simulink library "AtomicLibrary"
PostLoadFcn:
  | PacketBusGenerator
libraries: LinkLayer5 x2

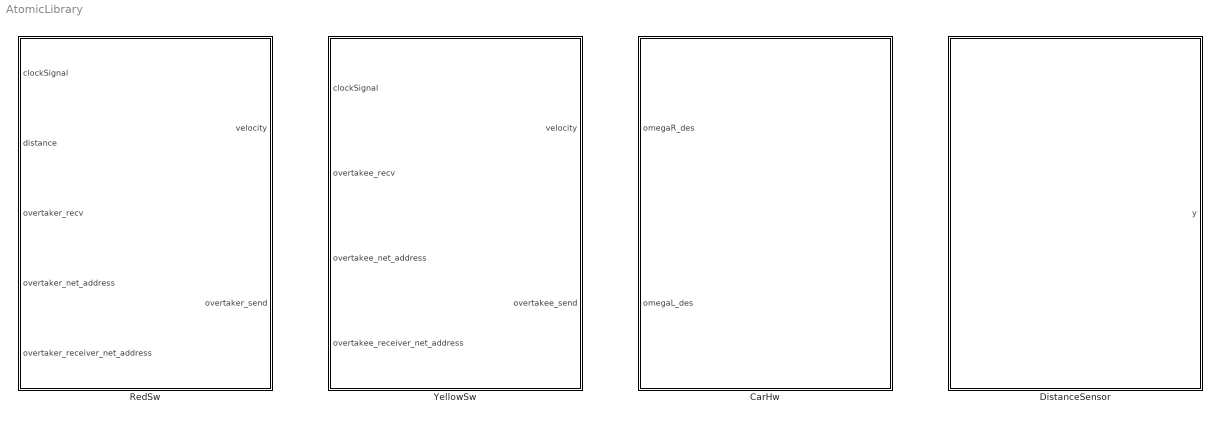
== system AtomicLibrary ==
  RedSw : Subsystem  Tag=id=_73wJYPUnEeOqvInL61-gjw
  YellowSw : Subsystem  Tag=id=_74DEU_UnEeOqvInL61-gjw
  CarHw : Subsystem  Tag=id=_74WmUPUnEeOqvInL61-gjw
  DistanceSensor : Subsystem  Tag=id=_74WmUfUnEeOqvInL61-gjw

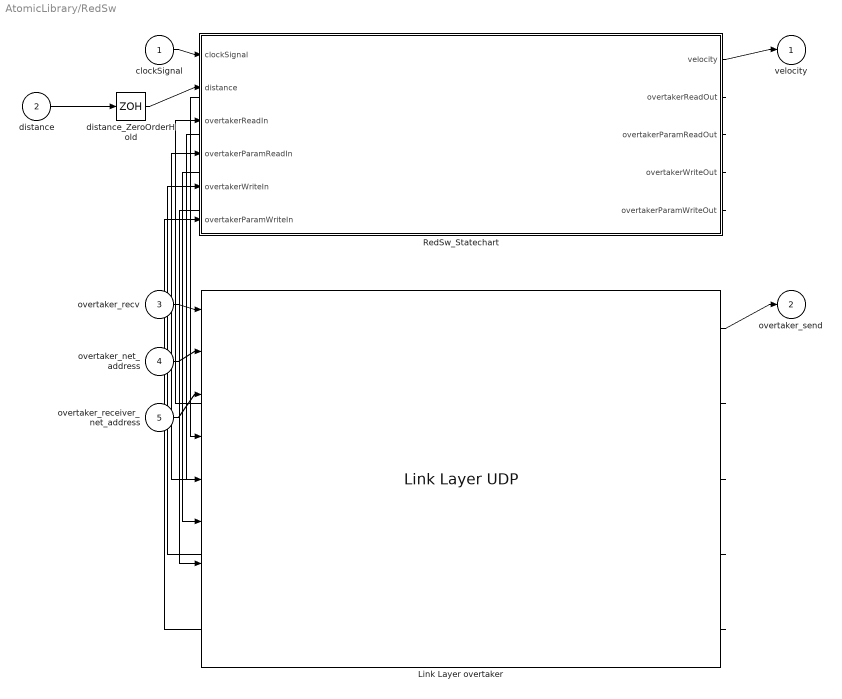
== system AtomicLibrary/RedSw ==
  clockSignal : Inport  Tag=id=_7356YvUnEeOqvInL61-gjw  Port=1  DataType=auto  OutDataType=fixdt(1, 16)  OutScaling=2^0  OutDataTypeStr=Inherit: auto
  distance : Inport  Tag=id=_77xGsPUnEeOqvInL61-gjw  Port=2  DataType=double  OutDataType=fixdt(1, 16)  OutScaling=2^0  OutDataTypeStr=double
  overtaker_recv : Inport  Tag=id=_780PkfUnEeOqvInL61-gjw  Port=3  DataType=auto  OutDataType=fixdt(1, 16)  OutScaling=2^0  UseBusObject=on  OutDataTypeStr=Inherit: auto
      settings: BusObject=PacketBus
  overtaker_net_address : Inport  Tag=id=_780Pk_UnEeOqvInL61-gjw  Port=4  DataType=uint8  OutDataType=fixdt(1, 16)  OutScaling=2^0  OutDataTypeStr=uint8
  overtaker_receiver_net_address : Inport  Tag=id=_780PlPUnEeOqvInL61-gjw  Port=5  DataType=uint8  OutDataType=fixdt(1, 16)  OutScaling=2^0  OutDataTypeStr=uint8
  velocity : Outport  Tag=id=_77VB0vUnEeOqvInL61-gjw  Port=1  DataType=double  OutDataType=fixdt(1, 16)  OutScaling=2^0  OutDataTypeStr=double
  overtaker_send : Outport  Tag=id=_780PkPUnEeOqvInL61-gjw  Port=2  DataType=auto  OutDataType=fixdt(1, 16)  OutScaling=2^0  UseBusObject=on  OutDataTypeStr=Inherit: auto
      settings: BusObject=PacketBus
  RedSw_Statechart : Stateflow chart  Tag=id=_73m_cPUnEeOqvInL61-gjw
  distance_ZeroOrderHold : ZeroOrderHold  Tag=id=_7763sPUnEeOqvInL61-gjw  SampleTime=30*0.001*1
  Link Layer overtaker : LinkLayer5/Link Layer UDP  DelayMin=1*1000  DelayMax=1*1000  MessageLossProbability=0  BufferOverflowPossible=on  SourceBufferSize=5  MessageMapping=[1 1; 2 1; 3 1; 4 1; 5 1]
  wires:
  clockSignal/1 -> RedSw_Statechart/1(clockSignal)
  RedSw_Statechart/1(velocity) -> velocity/1
  distance/1 -> distance_ZeroOrderHold/1
  distance_ZeroOrderHold/1 -> RedSw_Statechart/2(distance)
  Link Layer overtaker/1 -> overtaker_send/1
  overtaker_recv/1 -> Link Layer overtaker/1
  overtaker_net_address/1 -> Link Layer overtaker/2
  overtaker_receiver_net_address/1 -> Link Layer overtaker/3
  RedSw_Statechart/2(overtakerReadOut) -> Link Layer overtaker/4
  RedSw_Statechart/3(overtakerParamReadOut) -> Link Layer overtaker/5
  RedSw_Statechart/4(overtakerWriteOut) -> Link Layer overtaker/6
  RedSw_Statechart/5(overtakerParamWriteOut) -> Link Layer overtaker/7
  Link Layer overtaker/2 -> RedSw_Statechart/3(overtakerReadIn)
  Link Layer overtaker/3 -> RedSw_Statechart/4(overtakerParamReadIn)
  Link Layer overtaker/4 -> RedSw_Statechart/5(overtakerWriteIn)
  Link Layer overtaker/5 -> RedSw_Statechart/6(overtakerParamWriteIn)

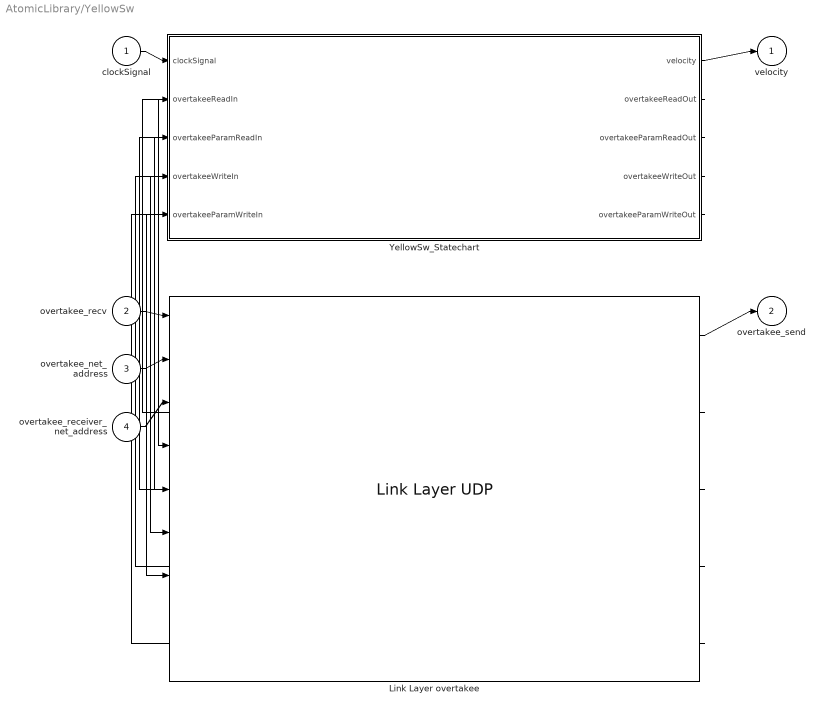
== system AtomicLibrary/YellowSw ==
  clockSignal : Inport  Tag=id=_74DEVvUnEeOqvInL61-gjw  Port=1  DataType=auto  OutDataType=fixdt(1, 16)  OutScaling=2^0  OutDataTypeStr=Inherit: auto
  overtakee_recv : Inport  Tag=id=_78gtlvUnEeOqvInL61-gjw  Port=2  DataType=auto  OutDataType=fixdt(1, 16)  OutScaling=2^0  UseBusObject=on  OutDataTypeStr=Inherit: auto
      settings: BusObject=PacketBus
  overtakee_net_address : Inport  Tag=id=_78gtmPUnEeOqvInL61-gjw  Port=3  DataType=uint8  OutDataType=fixdt(1, 16)  OutScaling=2^0  OutDataTypeStr=uint8
  overtakee_receiver_net_address : Inport  Tag=id=_78gtmfUnEeOqvInL61-gjw  Port=4  DataType=uint8  OutDataType=fixdt(1, 16)  OutScaling=2^0  OutDataTypeStr=uint8
  velocity : Outport  Tag=id=_77Bf0vUnEeOqvInL61-gjw  Port=1  DataType=double  OutDataType=fixdt(1, 16)  OutScaling=2^0  OutDataTypeStr=double
  overtakee_send : Outport  Tag=id=_78gtlfUnEeOqvInL61-gjw  Port=2  DataType=auto  OutDataType=fixdt(1, 16)  OutScaling=2^0  UseBusObject=on  OutDataTypeStr=Inherit: auto
      settings: BusObject=PacketBus
  YellowSw_Statechart : Stateflow chart  Tag=id=_74DEUfUnEeOqvInL61-gjw
  Link Layer overtakee : LinkLayer5/Link Layer UDP  DelayMin=1*1000  DelayMax=1*1000  MessageLossProbability=0  BufferOverflowPossible=on  SourceBufferSize=5  MessageMapping=[1 1; 2 1; 3 1; 4 1; 5 1]
  wires:
  clockSignal/1 -> YellowSw_Statechart/1(clockSignal)
  YellowSw_Statechart/1(velocity) -> velocity/1
  Link Layer overtakee/1 -> overtakee_send/1
  overtakee_recv/1 -> Link Layer overtakee/1
  overtakee_net_address/1 -> Link Layer overtakee/2
  overtakee_receiver_net_address/1 -> Link Layer overtakee/3
  YellowSw_Statechart/2(overtakeeReadOut) -> Link Layer overtakee/4
  YellowSw_Statechart/3(overtakeeParamReadOut) -> Link Layer overtakee/5
  YellowSw_Statechart/4(overtakeeWriteOut) -> Link Layer overtakee/6
  YellowSw_Statechart/5(overtakeeParamWriteOut) -> Link Layer overtakee/7
  Link Layer overtakee/2 -> YellowSw_Statechart/2(overtakeeReadIn)
  Link Layer overtakee/3 -> YellowSw_Statechart/3(overtakeeParamReadIn)
  Link Layer overtakee/4 -> YellowSw_Statechart/4(overtakeeWriteIn)
  Link Layer overtakee/5 -> YellowSw_Statechart/5(overtakeeParamWriteIn)

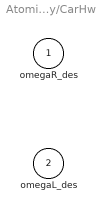
== system AtomicLibrary/CarHw ==
  omegaR_des : Inport  Tag=id=_76bp8PUnEeOqvInL61-gjw  Port=1  DataType=double  OutDataType=fixdt(1, 16)  OutScaling=2^0  OutDataTypeStr=double
  omegaL_des : Inport  Tag=id=_76la8PUnEeOqvInL61-gjw  Port=2  DataType=double  OutDataType=fixdt(1, 16)  OutScaling=2^0  OutDataTypeStr=double

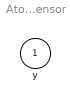
== system AtomicLibrary/DistanceSensor ==
  y : Outport  Tag=id=_764V4PUnEeOqvInL61-gjw  Port=1  DataType=double  OutDataType=fixdt(1, 16)  OutScaling=2^0  OutDataTypeStr=double

== stateflow chart YellowSw/YellowSw_Statechart ==
  state chart
    state chartRegion [parallel]
      settings: executionOrder=2
      state yellowSW_Component_Main
        state overtakee
          state noAcceleration
            state overtakee_noAcceleration
              state noBraking
              state brakingAllowed
              noBraking -> brakingAllowed : [overtakee_checkQueue(EVT_LANECHANGED, overtakeeReadOut)]
                  | {[overtakeeReadOut, overtakeeParamReadOut] = overtakee_dequeue(EVT_LANECHANGED, overtakeeReadOut, overtakeeParamReadOut); }
          state noOvertaking
            entry: localVelocity = 2 ;  velocity = localVelocity;
            state overtakee_noOvertaking
              state init
              state received
                entry: c2=reset();
              state Inv_Error
                entry: invariant();
              init -> received : [overtakee_checkQueue(EVT_REQUEST, overtakeeReadOut)]
                  | {[overtakeeReadOut, overtakeeParamReadOut] = overtakee_dequeue(EVT_REQUEST, overtakeeReadOut, overtakeeParamReadOut); }
              received -> init [order 2] : {[overtakeeWriteOut, overtakeeParamWriteOut] = overtakee_enqueue(EVT_DECLINE_FRONTVELOCITY, overtakeeWriteOut, double(localVelocity), overtakeeParamWriteOut)
                  | ; }
              received -> Inv_Error [order 3] : [time(c2) > 3*1000]
          noAcceleration -> noOvertaking : [overtakee_checkQueue(EVT_FINISH, overtakeeReadOut)]
              | {[overtakeeReadOut, overtakeeParamReadOut] = overtakee_dequeue(EVT_FINISH, overtakeeReadOut, overtakeeParamReadOut); }
    state DataInit [parallel]
      settings: executionOrder=1
    DataInit -> DataInit : {overtakeeWriteOut = overtakeeWriteIn;
        | overtakeeParamWriteOut = overtakeeParamWriteIn;
        | overtakeeReadOut = overtakeeReadIn;
        | overtakeeParamReadOut = overtakeeParamReadIn;
        | ; }
  (default) -> noBraking
  (default) -> init
  (default) -> noOvertaking
  (default) -> yellowSW_Component_Main
  (default) -> chart
  data: c2 local double =0.0; localVelocity local int32 =0; clock function_input double; logicalTime function_output uint32; clock function_output double; event function_input uint8; evtQueueIn function_input uint8 size=[5]; param function_input double; paramQueueIn function_input double size=[5]; evtQueue function_output uint8 size=[5]; paramQueue function_output double size=[5]; event function_input uint8; evtQueueIn function_input uint8 size=[5]; paramQueueIn function_input double size=[5]; evtQueue function_output uint8 size=[5]; paramQueue function_output double size=[5]; parameter function_output double; event function_input uint8; evtQueue function_input uint8 size=[5]; available function_output boolean; clockSignal input double; overtakeeReadIn input uint8 size=[5]; overtakeeParamReadIn input double size=5; overtakeeWriteIn input uint8 size=[5]; overtakeeParamWriteIn input double size=5; velocity output double = 0; overtakeeReadOut output uint8 size=[5]; overtakeeParamReadOut output double size=5; overtakeeWriteOut output uint8 size=[5]; overtakeeParamWriteOut output double size=5; EVT_DECLINE_FRONTVELOCITY constant uint32 =3; EVT_ACCEPT constant uint32 =2; EVT_REQUEST constant uint32 =1; EVT_FINISH constant uint32 =4; EVT_LANECHANGED constant uint32 =5
  function logicalTime = time(clock):
    | function logicalTime = time(clock) 
    | 
    |  sample = 0.001;  % the sample time of the system clock 
    | 
    |  %convert to pass units of time after last reset 
    | 
    |  logicalTime = uint32((clockSignal - clock)/sample);
  function clock = reset():
    | function clock = reset() 
    | 
    |  %set clock variable to current time 
    | 
    |  clock = clockSignal;
  function invariant():
    | function invariant() 
    |  error('Simulation stopped in Error State. An invariant is violated');
  function [evtQueue, paramQueue] = overtakee_enqueue(event, evtQueueIn, param, paramQueueIn):
    | function [evtQueue, paramQueue] = overtakee_enqueue(event, evtQueueIn, param, paramQueueIn) %eml 
    |  evtQueue = evtQueueIn; 
    |  paramQueue = paramQueueIn; 
    |  for i = 1:length(evtQueue) 
    |  	if evtQueue(i) == uint8(0) 
    |  		evtQueue(i) = event; 
    |  		paramQueue(i) = param; 
    |  		return 
    |  	end 
    |  end
  function [evtQueue, paramQueue, parameter] = overtakee_dequeue(event, evtQueueIn, paramQueueIn):
    | function [evtQueue, paramQueue, parameter] = overtakee_dequeue(event, evtQueueIn, paramQueueIn) %eml 
    |   evtQueue = evtQueueIn; 
    |   paramQueue = paramQueueIn; 
    |   parameter = 0; 
    |   for i = 1:length(evtQueue) 
    |     if evtQueue(i) == event 
    |          parameter = paramQueue(i); 
    |          for j = i:length(evtQueue)-1 
    |              evtQueue(j) = evtQueue(j+1); 
    |              paramQueue(j) = paramQueue(j+1); 
    |          end 
    |          evtQueue(length(evtQueue)) = 0;
    |          paramQueue(length(paramQueue)) = 0; 
    |          return 
    |      end 
    |   end
  function available = overtakee_checkQueue(event, evtQueue):
    | function available = overtakee_checkQueue(event, evtQueue) %eml 
    |  available = false; 
    |  for i = 1:length(evtQueue) 
    |      if evtQueue(i) == event 
    |          available = true;    
    |          return 
    |      end 
    |  end

== stateflow chart RedSw/RedSw_Statechart ==
  state chart
    state chartRegion [parallel]
      settings: executionOrder=2
      state redSW_Component_Main
        state overtaker
          state overtaking
            entry: c1=reset();
            state overtaker_overtaking
              state init
              state changed
              chart.chartRegion.redSW_Component_Main.overtaker.overtaking.overtaker_overtaking.init -> changed : {[overtakerWriteOut, overtakerParamWriteOut] = overtaker_enqueue(EVT_LANECHANGED, overtakerWriteOut, 0, overtakerParamWriteOut); }
          state noOvertaking
            entry: velocity = 8;
            state overtaker_noOvertaking
              state init
              state requested
                entry: c1=reset();
              state Wait
              state Inv_Error
                entry: invariant();
              chart.chartRegion.redSW_Component_Main.overtaker.noOvertaking.overtaker_noOvertaking.init -> requested : [distance < 0.1]
                  | {[overtakerWriteOut, overtakerParamWriteOut] = overtaker_enqueue(EVT_REQUEST, overtakerWriteOut, 0, overtakerParamWriteOut); }
              requested -> chart.chartRegion.redSW_Component_Main.overtaker.noOvertaking.overtaker_noOvertaking.init [order 2] : [time(c1) >= 6*1000]
              requested -> Wait [order 3] : [overtaker_checkQueue(EVT_DECLINE_FRONTVELOCITY, overtakerReadOut)]
                  | {c2=reset(); velocity = tmp_var_1; [overtakerReadOut, overtakerParamReadOut, tmp_var_1] = overtaker_dequeue(EVT_DECLINE_FRONTVELOCITY, overtakerReadOut, overtakerParamReadOut); }
              Wait -> chart.chartRegion.redSW_Component_Main.overtaker.noOvertaking.overtaker_noOvertaking.init : [time(c2) > 2*1000]
              requested -> chart.chartRegion.redSW_Component_Main.overtaker.noOvertaking.overtaker_noOvertaking.Inv_Error [order 4] : [time(c1) > 7*1000]
          state Inv_Error
            entry: invariant();
          overtaking -> chart.chartRegion.redSW_Component_Main.overtaker.Inv_Error : [time(c1) > 10*1000]
    state DataInit [parallel]
      settings: executionOrder=1
    DataInit -> DataInit : {overtakerWriteOut = overtakerWriteIn;
        | overtakerParamWriteOut = overtakerParamWriteIn;
        | overtakerReadOut = overtakerReadIn;
        | overtakerParamReadOut = overtakerParamReadIn;
        | ; }
  (default) -> chart.chartRegion.redSW_Component_Main.overtaker.overtaking.overtaker_overtaking.init
  (default) -> chart.chartRegion.redSW_Component_Main.overtaker.noOvertaking.overtaker_noOvertaking.init
  (default) -> noOvertaking
  (default) -> redSW_Component_Main
  (default) -> chart
  data: c1 local double =0.0; c2 local double =0.0; clock function_input double; logicalTime function_output uint32; clock function_output double; event function_input uint8; evtQueueIn function_input uint8 size=[5]; param function_input double; paramQueueIn function_input double size=[5]; evtQueue function_output uint8 size=[5]; paramQueue function_output double size=[5]; event function_input uint8; evtQueueIn function_input uint8 size=[5]; paramQueueIn function_input double size=[5]; evtQueue function_output uint8 size=[5]; paramQueue function_output double size=[5]; parameter function_output double; event function_input uint8; evtQueue function_input uint8 size=[5]; available function_output boolean; clockSignal input double; distance input double; overtakerReadIn input uint8 size=[5]; overtakerParamReadIn input double size=5; overtakerWriteIn input uint8 size=[5]; overtakerParamWriteIn input double size=5; velocity output double; overtakerReadOut output uint8 size=[5]; overtakerParamReadOut output double size=5; overtakerWriteOut output uint8 size=[5]; overtakerParamWriteOut output double size=5; EVT_DECLINE_FRONTVELOCITY constant uint32 =3; EVT_REQUEST constant uint32 =1; EVT_FINISH constant uint32 =4; EVT_LANECHANGED constant uint32 =5; EVT_ACCEPT constant uint32 =2; tmp_var_1 local double
  function logicalTime = time(clock):
    | function logicalTime = time(clock) 
    | 
    |  sample = 0.001;  % the sample time of the system clock 
    | 
    |  %convert to pass units of time after last reset 
    | 
    |  logicalTime = uint32((clockSignal - clock)/sample);
  function clock = reset():
    | function clock = reset() 
    | 
    |  %set clock variable to current time 
    | 
    |  clock = clockSignal;
  function invariant():
    | function invariant() 
    |  error('Simulation stopped in Error State. An invariant is violated');
  function [evtQueue, paramQueue] = overtaker_enqueue(event, evtQueueIn, param, paramQueueIn):
    | function [evtQueue, paramQueue] = overtaker_enqueue(event, evtQueueIn, param, paramQueueIn) %eml 
    |  evtQueue = evtQueueIn; 
    |  paramQueue = paramQueueIn; 
    |  for i = 1:length(evtQueue) 
    |  	if evtQueue(i) == uint8(0) 
    |  		evtQueue(i) = event; 
    |  		paramQueue(i) = param; 
    |  		return 
    |  	end 
    |  end
  function [evtQueue, paramQueue, parameter] = overtaker_dequeue(event, evtQueueIn, paramQueueIn):
    | function [evtQueue, paramQueue, parameter] = overtaker_dequeue(event, evtQueueIn, paramQueueIn) %eml 
    |   evtQueue = evtQueueIn; 
    |   paramQueue = paramQueueIn; 
    |   parameter = 0; 
    |   for i = 1:length(evtQueue) 
    |     if evtQueue(i) == event 
    |          parameter = paramQueue(i); 
    |          for j = i:length(evtQueue)-1 
    |              evtQueue(j) = evtQueue(j+1); 
    |              paramQueue(j) = paramQueue(j+1); 
    |          end 
    |          evtQueue(length(evtQueue)) = 0;
    |          paramQueue(length(paramQueue)) = 0; 
    |          return 
    |      end 
    |   end
  function available = overtaker_checkQueue(event, evtQueue):
    | function available = overtaker_checkQueue(event, evtQueue) %eml 
    |  available = false; 
    |  for i = 1:length(evtQueue) 
    |      if evtQueue(i) == event 
    |          available = true;    
    |          return 
    |      end 
    |  end
